simulink model "step2f"  (Simulink 8.5)
settings: Solver=ode45  SolverMode=SingleTasking  StartTime=0.0  StopTime=0.099  MaxStep=1e-4  RelTol=1e-4  AbsTol=1e-6
undefined symbols (not defined in the file or in its folder): den, dx, num
libraries: elements x1
settings Model: Creator=PC  LastModifiedBy=PC  ExtModeTrigMode=oneshot  ExtModeArmWhenConnect=off
settings DataIOCC: LimitDataPoints=off
settings OptimizationCC: BlockReduction=off  BooleanDataType=off  ExpressionDepthLimit=128
settings DebuggingCC: SaveWithParameterizedLinksMsg=none  SignalResolutionControl=TryResolveAllWithWarning  MultiTaskDSMMsg=warning  MultiTaskCondExecSysMsg=none  FcnCallInpInsideContextMsg=EnableAllAsError  StateNameClashWarn=none  StrictBusMsg=None
settings HardwareCC: TargetUnknown=on
settings RTWCC: TemplateMakefile=grt_vc.tmf

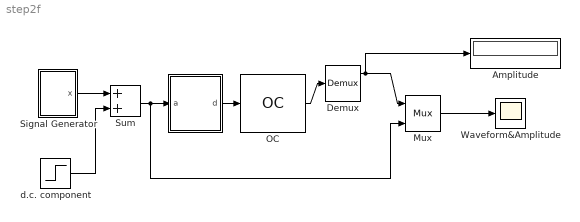
== system step2f ==
  "  " : Subsystem  mask(Data Adquisition Board){filter=on, approx=Butterworth, order=3, numerator=[], denominator=[], freq=180, resdis=on, vertres=8, xmax=100, winsize=20, G=1.0, fs=60*20}
      mask prompts: filter "Disable Analog Filter"; approx "Filter approximation"; numerator "Free expression filter: numerator(descending order of s)"; denominator "Free expression filter: denominator:"; freq "Cut-off frequency"; resdis "Disable Vertical Resolution"; vertres "Vertical Resolution: No. of bits"; xmax "Vertical Resolution: signal range"; winsize "Window size"; G "Gain"; fs "Sampling frequency"
      mask help: Takes the instantaneous value of the input signal and convert it to the data window of samples.
      mask init:
      | dab1
      mask TypeOptions approx: Bessel | Tschebyscheff | Butterworth | free expression
      mask TypeOptions order: 2 | 3 | 4
      mask TypeOptions vertres: 8 | 12 | 16
      mask Display: disp('DAB')
  Amplitude : Display
  Demux : Demux  Outputs=2
  Mux : Mux  Inputs=2
  OC : elements/OC  tfilt=Fourier  rfilt=[ ]  ifilt=[ ]  tlen=full  N1=20
  Signal Generator : Subsystem  mask(Signal Generator){A1=1, f1=60, A2=0, f2=2*60, A3=0, f3=5*60, tstart=1.5/60}
      mask prompts: A1 "Amplitude 1"; f1 "Frequency 1 [Hz]"; A2 "Amplitude 2"; f2 "Frequency 2 [Hz]"; A3 "Amplitude 3"; f3 "Frequency 3 [Hz]"; tstart "Start time [sec]"
  Sum : Sum  SaturateOnIntegerOverflow=on  InputSameDT=on  OutDataTypeStr=Inherit: Same as first input
  Waveform&Amplitude : Scope
      settings: TickLabels=on  YMin=-1.2  YMax=2
  d.c. component : Step  Time=1.5/60  After=0.5
  wires:
  Sum/1 -> Mux/2, "  "/1(a)
  d.c. component/1 -> Sum/2
  Signal Generator/1(x) -> Sum/1
  Mux/1 -> Waveform&Amplitude/1
  Demux/1 -> Mux/1, Amplitude/1
  OC/1 -> Demux/1
  "  "/1(d) -> OC/1

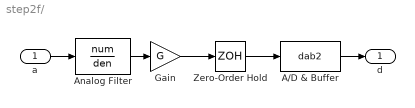
== system step2f/   ==
  a : Inport
  A/D & Buffer : S-Function  FunctionName=dab2  Parameters=winsize,fs,dx,resdis
  Analog Filter : TransferFcn  Numerator=num  Denominator=den
  Gain : Gain  Gain=G  SaturateOnIntegerOverflow=on  OutDataTypeStr=Inherit: Same as input  ParamDataTypeStr=Inherit: Same as input
  Zero-Order Hold : ZeroOrderHold  SampleTime=1/fs
  d : Outport  InitialOutput=[zeros(winsize,1)]
  wires:
  Analog Filter/1 -> Gain/1
  Gain/1 -> Zero-Order Hold/1
  Zero-Order Hold/1 -> A/D & Buffer/1
  a/1 -> Analog Filter/1
  A/D & Buffer/1 -> d/1

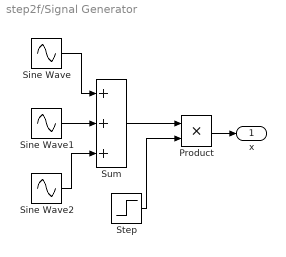
== system step2f/Signal Generator ==
  Product : Product  SaturateOnIntegerOverflow=on  RndMeth=Zero  InputSameDT=on  OutDataTypeStr=Inherit: Same as first input
  Sine Wave : Sin  Amplitude=A1  Frequency=f1*2*pi  SampleTime=0
  Sine Wave1 : Sin  Amplitude=A2  Frequency=f2*2*pi  SampleTime=0
  Sine Wave2 : Sin  Amplitude=A3  Frequency=f3*2*pi  SampleTime=0
  Step : Step  Time=tstart
  Sum : Sum  Inputs=+++  SaturateOnIntegerOverflow=on  InputSameDT=on  OutDataTypeStr=Inherit: Same as first input
  x : Outport  InitialOutput=0
  wires:
  Sine Wave/1 -> Sum/1
  Sine Wave1/1 -> Sum/2
  Sine Wave2/1 -> Sum/3
  Sum/1 -> Product/1
  Step/1 -> Product/2
  Product/1 -> x/1
